simulink model "Base"  (R2013b)
settings: Solver=ode23t  StartTime=0.0  StopTime=1  RelTol=1e-3
undefined symbols (not defined in the file): DiscIntNeverNeededParam
libraries: nesl_utility x11, pe_lib x10, fl_lib x7
Description:
  | Three-Phase PMSM Drive
  | 
  | This example shows a Permanent Magnet Synchronous Machine
  | (PMSM) and inverter sized for use in a typical hybrid vehicle.
  | Here the inverter is connected directly to the vehicle battery, but
  | often there is also a DC-DC converter stage in between. The
  | model can be used to design the PMSM controller, selecting
  | architecture and gains to achieve desired performance. To check
  | the timing of IGBT turn-on and turn-off, the IGBT devices can be
  | directly replaced by more detailed device models from
  | SimElectronics(TM). For complete vehicle modeling, the
  | SimElectronics(R) Servomotor block can be used to abstract the
  | PMSM, inverter and controller with an energy-based model.
  | The Gmin resistor provides a very small conductance to ground
  | that improves the numerical properties of the model when using
  | a variable-step solver.
  | 
  | 
  | Copyright 2008-2013 The MathWorks, Inc.
settings Model: Creator=MathWorks  LastModifiedBy=Eduardo
settings DebuggingCC: SolverPrmCheckMsg=none

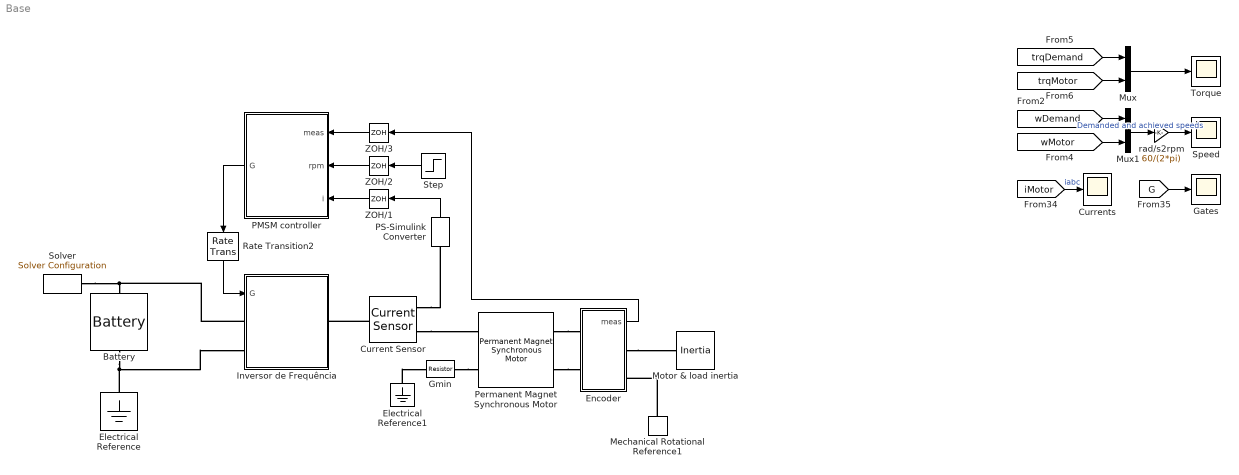
== system Base ==
  Battery : pe_lib/Sources/Battery  Vnom=500 V  AH=14000 hr*A  AH0=7000 hr*A  V1=470 V  AH1=5000 hr*A  R1=0.001 Ohm  R2=inf Ohm  alpha=1  beta=1  G2=0 S  i_Log=off  charge_Log=off  LocalVarNames=|i|charge  LocalVarDescs=|i|Charge state  LocalVarLogging=[0 0]
  Current Sensor : pe_lib/Sensors/Current Sensor  I_Log=off  LocalVarNames=|i_a|i_b|i_c  LocalVarDescs=|i_a|i_b|i_c  LocalVarLogging=[0 0 0]  i_a_Log=off  i_b_Log=off  i_c_Log=off
  Currents : Scope
      settings: TimeRange=1  YMin=-2200  YMax=2200  SaveName=ScopeData5  MaxDataPoints=50000  Decimation=10
  Electrical Reference : fl_lib/Electrical/Electrical Elements/Electrical Reference  i_Log=off  LocalVarNames=|i  LocalVarDescs=|i  LocalVarLogging=0
  Electrical Reference1 : fl_lib/Electrical/Electrical Elements/Electrical Reference  i_Log=off  LocalVarNames=|i  LocalVarDescs=|i  LocalVarLogging=0
  Encoder : Subsystem
  Gates : Scope
      settings: TimeRange=0.01  YMin=-0.1  YMax=1.1  SaveName=ScopeData4  MaxDataPoints=50000  Decimation=10
  Gmin : fl_lib/Electrical/Electrical Elements/Resistor  R=1e9 Ohm  i_Log=off  v_Log=off  LocalVarNames=|i|v  LocalVarDescs=|i|v  LocalVarLogging=[0 0]
  Inversor de Frequência : Subsystem
  Mechanical Rotational Reference1 : fl_lib/Mechanical/Rotational Elements/Mechanical Rotational Reference  t_Log=off  LocalVarNames=|t  LocalVarDescs=|t  LocalVarLogging=0
  Motor & load inertia : fl_lib/Mechanical/Rotational Elements/Inertia  inertia=10 kg*m^2  initial_velocity=0 rpm  t_Log=off  LocalVarNames=|t  LocalVarDescs=|t  LocalVarLogging=0
  Mux : Mux  Inputs=2
  Mux1 : Mux  Inputs=2
  PMSM controller : Subsystem
  PS-Simulink Converter : nesl_utility/PS-Simulink Converter  PhysicalDomain=network_engine_domain  SubClassName=ps_output  LeftPortType=input  RightPortType=output  PseudoPeriodic=off  Frequencies=[]  Unit=A  AffineConversion=off
  Permanent Magnet Synchronous Motor : pe_lib/Machines/Permanent Magnet Rotor/Permanent Magnet Synchronous Motor  nPolePairs=8  pm_flux_linkage=0.03 Wb  stator_param=1  Ld=0.00025 H  Lq=0.00019 H  L0=0.00016 H  Ls=0.0002 H  Lm=0 H  Ms=0 H  Rs=0.013 Ohm  initial_currents=[0, 0, 0] A  axes_param=1  angular_position0=0 deg  LocalVarNames=|i_d|i_q|i_0|v_a|v_b|v_c|i_a|i_b|i_c|torque|angular_velocity|angular_position  LocalVarDescs=|i_d|i_q|i_0|v_a|v_b|v_c|i_a|i_b|i_c|torque|angular_velocity|angular_position  LocalVarLogging=[0 0 0 0 0 0 0 0 0 0 0 0]  rotor_offset=- pi / 2 rad  shift_3ph=[nan, nan, nan] rad  sqrt2OverSqrt3=nan  oneOverSqrt2=nan  twoPiOver3=nan  Lmin=1e-9 H  i_d_Log=off  i_q_Log=off  i_0_Log=off  v_a_Log=off  v_b_Log=off  v_c_Log=off  i_a_Log=off  i_b_Log=off  i_c_Log=off  i_n_Log=off  torque_Log=off  angular_velocity_Log=off  angular_position_Log=off
  Rate Transition2 : RateTransition
  Solver : nesl_utility/Solver Configuration  PhysicalDomain=network_engine_domain  SubClassName=solver  LeftPortType=input  RightPortType=generic  Accelerate=off  Tones=[]  Harmonics=[]  SimulateNoise=off  Profile=off  UseLocalSampling=off  EnableSwitchedLinearOptims=on  FrequencyDomain=off  UseCCode=off  RelTol=0.001  AbsTol=1e-06  MinStep=1e-09  ToWorkspace=off  DoDC=off  ResidualTolerance=1e-9  UseLocalSolver=on  LocalSolverChoice=NE_BACKWARD_EULER_ADVANCER  LocalSolverSampleTime=1e-5  DoFixedCost=on  MaxNonlinIter=3  MaxModeIter=2  LinearAlgebra=Sparse  DelaysMemoryBudget=1024
  Speed : Scope
      settings: YMin=-10  YMax=210  SaveName=ScopeData6  MaxDataPoints=50000  Decimation=10
  Step : Step  Time=0.1  After=200  SampleTime=0
  Torque : Scope
      settings: YMin=-100  YMax=600  SaveName=ScopeData7  MaxDataPoints=50000  Decimation=10
  ZOH/1 : ZeroOrderHold  SampleTime=1e-4
  ZOH/2 : ZeroOrderHold  SampleTime=1e-2
  ZOH/3 : ZeroOrderHold  SampleTime=1e-4
  rad/s2rpm : Gain  Gain=60/(2*pi)
  wires:
  Step/1 -> ZOH/2/1
  PS-Simulink Converter/1 -> ZOH/1/1
  PMSM controller/1(G) -> Rate Transition2/1
  rad/s2rpm/1 -> Speed/1
  [iMotor] -> Currents/1  "iabc"
  [G] -> Gates/1
  Mux1/1 -> rad/s2rpm/1  "Demanded and achieved speeds"
  [wMotor] -> Mux1/2
  [wDemand] -> Mux1/1
  Mux/1 -> Torque/1
  [trqMotor] -> Mux/2
  [trqDemand] -> Mux/1
  ZOH/1/1 -> PMSM controller/3(i)
  ZOH/2/1 -> PMSM controller/2(rpm)
  Encoder/1(meas) -> ZOH/3/1
  ZOH/3/1 -> PMSM controller/1(meas)
  Rate Transition2/1 -> Inversor de Frequência/1(G)
  connections:
  Permanent Magnet Synchronous Motor/RConn1 -- Encoder/LConn1
  Permanent Magnet Synchronous Motor/RConn2 -- Encoder/LConn2
  Encoder/RConn1 -- Motor & load inertia/LConn1
  Mechanical Rotational Reference1/LConn1 -- Encoder/RConn2
  Current Sensor/LConn1 -- Inversor de Frequência/RConn1
  Battery/RConn1 -- Inversor de Frequência/LConn2 -- Electrical Reference/LConn1
  Current Sensor/RConn2 -- Permanent Magnet Synchronous Motor/LConn1
  Current Sensor/RConn1 -- PS-Simulink Converter/LConn1
  Gmin/RConn1 -- Permanent Magnet Synchronous Motor/LConn2
  Electrical Reference1/LConn1 -- Gmin/LConn1
  Solver/RConn1 -- Inversor de Frequência/LConn1 -- Battery/LConn1

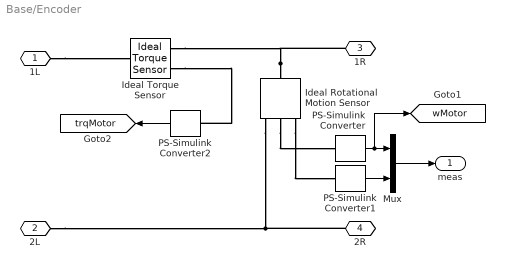
== system Base/Encoder ==
  Ideal Rotational Motion Sensor : fl_lib/Mechanical/Mechanical Sensors/Ideal Rotational Motion Sensor  offset=0 deg  w_Log=off  t_Log=off  phi_Log=off  LocalVarNames=|w|t|phi  LocalVarDescs=|w|t|phi  LocalVarLogging=[0 0 0]
  Ideal Torque Sensor : fl_lib/Mechanical/Mechanical Sensors/Ideal Torque Sensor  w_Log=off  t_Log=off  LocalVarNames=|w|t  LocalVarDescs=|w|t  LocalVarLogging=[0 0]
  Mux : Mux  Inputs=2
  PS-Simulink Converter : nesl_utility/PS-Simulink Converter  PhysicalDomain=network_engine_domain  SubClassName=ps_output  LeftPortType=input  RightPortType=output  PseudoPeriodic=off  Frequencies=[]  Unit=rad/s  AffineConversion=off
  PS-Simulink Converter1 : nesl_utility/PS-Simulink Converter  PhysicalDomain=network_engine_domain  SubClassName=ps_output  LeftPortType=input  RightPortType=output  PseudoPeriodic=off  Frequencies=[]  Unit=rad  AffineConversion=off
  PS-Simulink Converter2 : nesl_utility/PS-Simulink Converter  PhysicalDomain=network_engine_domain  SubClassName=ps_output  LeftPortType=input  RightPortType=output  PseudoPeriodic=off  Frequencies=[]  Unit=N*m  AffineConversion=off
  1L : PMIOPort  Port=1  Side=Left
  2L : PMIOPort  Port=2  Side=Left
  1R : PMIOPort  Port=3  Side=Right
  2R : PMIOPort  Port=4  Side=Right
  meas : Outport
  tag scope: trqMotor=global, wMotor=global
  wires:
  PS-Simulink Converter2/1 -> [trqMotor]
  Mux/1 -> meas/1
  PS-Simulink Converter1/1 -> Mux/2
  PS-Simulink Converter/1 -> [wMotor], Mux/1
  connections:
  Ideal Torque Sensor/RConn2 -- PS-Simulink Converter2/LConn1
  1L/RConn1 -- Ideal Torque Sensor/LConn1
  2R/RConn1 -- 2L/RConn1 -- Ideal Rotational Motion Sensor/RConn1
  Ideal Rotational Motion Sensor/LConn1 -- 1R/RConn1 -- Ideal Torque Sensor/RConn1
  Ideal Rotational Motion Sensor/RConn2 -- PS-Simulink Converter/LConn1
  Ideal Rotational Motion Sensor/RConn3 -- PS-Simulink Converter1/LConn1

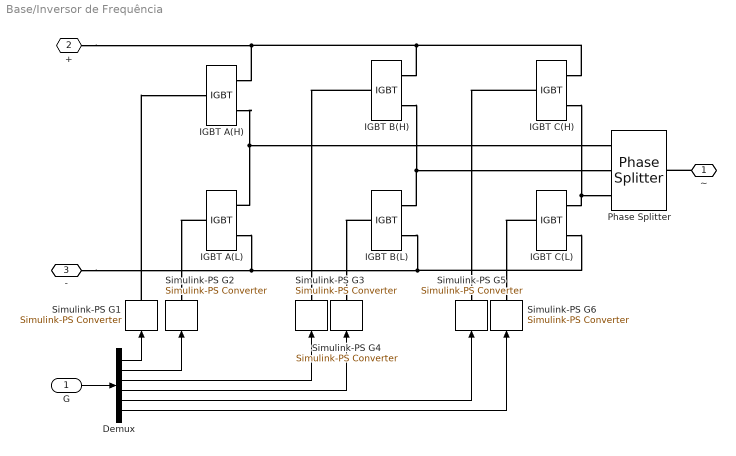
== system Base/Inversor de Frequência ==
  G : Inport
  Demux : Demux  Outputs=6
  IGBT A(H) : pe_lib/Semiconductors/Fundamental Components/IGBT  Vf=0.8 V  Ron=0.001 Ohm  Goff=1e-5 S  Vth=0.5 V  diode_param=2  diode_Vf=0.8 V  diode_Ron=0.001 Ohm  diode_Goff=1e-5 S  diode_C=5e-8 F  diode_iRM=-235 A  diode_iF=300 A  diode_idot=-50 A/us  diode_trr_param=1  diode_trr_factor=3  diode_trr=15 us  diode_Qrr=1.5e+3 s*uA  LocalVarLogging=[]
  IGBT A(L) : pe_lib/Semiconductors/Fundamental Components/IGBT  Vf=0.8 V  Ron=0.001 Ohm  Goff=1e-5 S  Vth=0.5 V  diode_param=2  diode_Vf=0.8 V  diode_Ron=0.001 Ohm  diode_Goff=1e-5 S  diode_C=5e-8 F  diode_iRM=-235 A  diode_iF=300 A  diode_idot=-50 A/us  diode_trr_param=1  diode_trr_factor=3  diode_trr=15 us  diode_Qrr=1.5e+3 s*uA  LocalVarLogging=[]
  IGBT B(H) : pe_lib/Semiconductors/Fundamental Components/IGBT  Vf=0.8 V  Ron=0.001 Ohm  Goff=1e-5 S  Vth=0.5 V  diode_param=2  diode_Vf=0.8 V  diode_Ron=0.001 Ohm  diode_Goff=1e-5 S  diode_C=5e-8 F  diode_iRM=-235 A  diode_iF=300 A  diode_idot=-50 A/us  diode_trr_param=1  diode_trr_factor=3  diode_trr=15 us  diode_Qrr=1.5e+3 s*uA  LocalVarLogging=[]
  IGBT B(L) : pe_lib/Semiconductors/Fundamental Components/IGBT  Vf=0.8 V  Ron=0.001 Ohm  Goff=1e-5 S  Vth=0.5 V  diode_param=2  diode_Vf=0.8 V  diode_Ron=0.001 Ohm  diode_Goff=1e-5 S  diode_C=5e-8 F  diode_iRM=-235 A  diode_iF=300 A  diode_idot=-50 A/us  diode_trr_param=1  diode_trr_factor=3  diode_trr=15 us  diode_Qrr=1.5e+3 s*uA  LocalVarLogging=[]
  IGBT C(H) : pe_lib/Semiconductors/Fundamental Components/IGBT  Vf=0.8 V  Ron=0.001 Ohm  Goff=1e-5 S  Vth=0.5 V  diode_param=2  diode_Vf=0.8 V  diode_Ron=0.001 Ohm  diode_Goff=1e-5 S  diode_C=5e-8 F  diode_iRM=-235 A  diode_iF=300 A  diode_idot=-50 A/us  diode_trr_param=1  diode_trr_factor=3  diode_trr=15 us  diode_Qrr=1.5e+3 s*uA  LocalVarLogging=[]
  IGBT C(L) : pe_lib/Semiconductors/Fundamental Components/IGBT  Vf=0.8 V  Ron=0.001 Ohm  Goff=1e-5 S  Vth=0.5 V  diode_param=2  diode_Vf=0.8 V  diode_Ron=0.001 Ohm  diode_Goff=1e-5 S  diode_C=5e-8 F  diode_iRM=-235 A  diode_iF=300 A  diode_idot=-50 A/us  diode_trr_param=1  diode_trr_factor=3  diode_trr=15 us  diode_Qrr=1.5e+3 s*uA  LocalVarLogging=[]
  Phase Splitter : pe_lib/Connections/Phase Splitter  I_Log=off  i_a_Log=off  i_b_Log=off  i_c_Log=off  LocalVarNames=|I|i_a|i_b|i_c  LocalVarDescs=|I|i_a|i_b|i_c  LocalVarLogging=[0 0 0 0]
  Simulink-PS G{1..6} (6 alike) : nesl_utility/Simulink-PS Converter  PhysicalDomain=network_engine_domain  SubClassName=ps_input  LeftPortType=input  RightPortType=output  PseudoPeriodic=off  Frequencies=[]  NoiseDistribution=none  NoiseParameters=[]  Unit=1  AffineConversion=off  InputFiltering=off  SimscapeFilterOrder=1  InputFilterTimeConstant=1e-6  UdotUserProvided=0
  ~ : PMIOPort  Tag=PMCPort  Port=1  Side=Right
  + : PMIOPort  Tag=PMCPort  Port=2  Side=Left
  - : PMIOPort  Tag=PMCPort  Port=3  Side=Left
  wires:
  Demux/6 -> Simulink-PS G6/1
  Demux/5 -> Simulink-PS G5/1
  Demux/4 -> Simulink-PS G4/1
  Demux/3 -> Simulink-PS G3/1
  Demux/2 -> Simulink-PS G2/1
  G/1 -> Demux/1
  Demux/1 -> Simulink-PS G1/1
  connections:
  IGBT C(L)/LConn1 -- Simulink-PS G6/RConn1
  IGBT C(H)/LConn1 -- Simulink-PS G5/RConn1
  IGBT B(L)/LConn1 -- Simulink-PS G4/RConn1
  IGBT B(H)/LConn1 -- Simulink-PS G3/RConn1
  IGBT A(L)/LConn1 -- Simulink-PS G2/RConn1
  -/RConn1 -- IGBT A(L)/RConn2 -- IGBT C(L)/RConn2 -- IGBT B(L)/RConn2
  IGBT A(H)/RConn2 -- IGBT A(L)/RConn1 -- Phase Splitter/RConn1
  IGBT B(L)/RConn1 -- IGBT B(H)/RConn2 -- Phase Splitter/RConn2
  IGBT C(L)/RConn1 -- IGBT C(H)/RConn2 -- Phase Splitter/RConn3
  +/RConn1 -- IGBT A(H)/RConn1 -- IGBT C(H)/RConn1 -- IGBT B(H)/RConn1
  ~/RConn1 -- Phase Splitter/LConn1
  Simulink-PS G1/RConn1 -- IGBT A(H)/LConn1

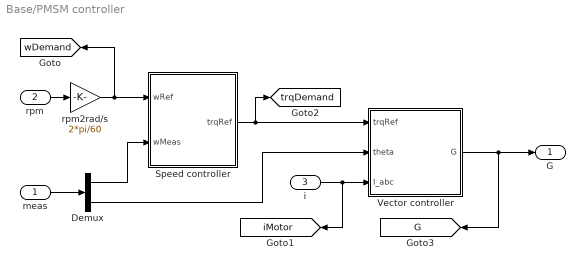
== system Base/PMSM controller ==
  meas : Inport
  rpm : Inport  Port=2
  i : Inport  Port=3
  Demux : Demux  Outputs=2
  Speed controller : Subsystem  mask(P+I motor speed controller){Kp=10000, Ki=10000, trqMax=500, ts=1e-2}
      mask prompts: Kp "Proportional gain (Nm/(rad/s))"; Ki "Integral gain (Nm/rad)"; trqMax "Maximum torque demand"; ts "Sample time"
      mask help: Inputs wRef and wMeas are the demanded rotor speed and measured rotor speed in rad/s. The controller output is a torque demand in Nm.
  Vector controller : Subsystem  mask(Vector controller){Np=6, lambda=0.03, h=1}
      mask prompts: Np "Number of pole pairs, p"; lambda "Flux linkage from rotor permanent magnet"; h "Current hysteresis (A)"
  rpm2rad/s : Gain  Gain=2*pi/60
  G : Outport
  tag scope: G=global, iMotor=global, trqDemand=global, wDemand=global
  wires:
  Vector controller/1(G) -> G/1, [G]
  Speed controller/1(trqRef) -> [trqDemand], Vector controller/1(trqRef)
  i/1 -> [iMotor], Vector controller/3(I_abc)
  rpm/1 -> rpm2rad/s/1
  rpm2rad/s/1 -> Speed controller/1(wRef), [wDemand]
  meas/1 -> Demux/1
  Demux/1 -> Speed controller/2(wMeas)
  Demux/2 -> Vector controller/2(theta)

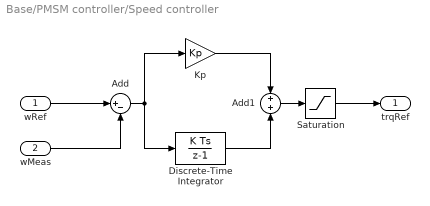
== system Base/PMSM controller/Speed controller ==
  wRef : Inport
  wMeas : Inport  Port=2
  Add : Sum  Inputs=|+-
  Add1 : Sum
  Discrete-Time Integrator : DiscreteIntegrator  gainval=Ki  SampleTime=ts  LimitOutput=on  UpperSaturationLimit=trqMax  LowerSaturationLimit=-trqMax  ICPrevOutput=DiscIntNeverNeededParam  ICPrevScaledInput=DiscIntNeverNeededParam
  Kp : Gain  Gain=Kp
  Saturation : Saturate  UpperLimit=trqMax  LowerLimit=-trqMax
  trqRef : Outport
  wires:
  wRef/1 -> Add/1
  Add1/1 -> Saturation/1
  Kp/1 -> Add1/1
  Discrete-Time Integrator/1 -> Add1/2
  wMeas/1 -> Add/2
  Saturation/1 -> trqRef/1
  Add/1 -> Kp/1, Discrete-Time Integrator/1

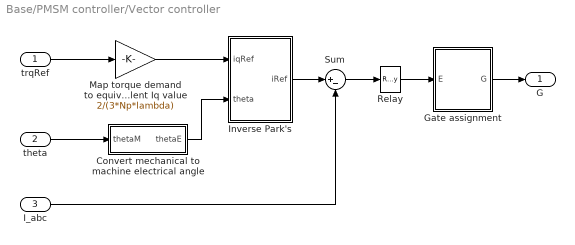
== system Base/PMSM controller/Vector controller ==
  trqRef : Inport
  theta : Inport  Port=2
  I_abc : Inport  Port=3
  Convert mechanical to machine electrical angle : Subsystem
  Gate assignment : Subsystem
  Inverse Park's : Subsystem
  Map torque demand to equivalent Iq value : Gain  Gain=2/(3*Np*lambda)  SaturateOnIntegerOverflow=on  OutDataTypeStr=Inherit: Same as input  ParamDataTypeStr=Inherit: Same as input
  Relay : Relay  OnSwitchValue=h/2  OffSwitchValue=-h/2
  Sum : Sum  Inputs=|+-  SaturateOnIntegerOverflow=on  InputSameDT=on  OutDataTypeStr=Inherit: Same as first input
  G : Outport
  wires:
  Convert mechanical to machine electrical angle/1(thetaE) -> Inverse Park's/2(theta)
  theta/1 -> Convert mechanical to machine electrical angle/1(thetaM)
  Map torque demand to equivalent Iq value/1 -> Inverse Park's/1(iqRef)
  I_abc/1 -> Sum/2
  trqRef/1 -> Map torque demand to equivalent Iq value/1
  Inverse Park's/1(iRef) -> Sum/1
  Sum/1 -> Relay/1
  Relay/1 -> Gate assignment/1(E)
  Gate assignment/1(G) -> G/1

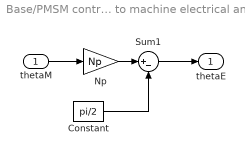
== system Base/PMSM controller/Vector controller/Convert mechanical to machine electrical angle ==
  thetaM : Inport
  Constant : Constant  Value=pi/2
  Np : Gain  Gain=Np  SaturateOnIntegerOverflow=on  OutDataTypeStr=Inherit: Same as input  ParamDataTypeStr=Inherit: Same as input
  Sum1 : Sum  Inputs=|+-
  thetaE : Outport
  wires:
  Constant/1 -> Sum1/2
  thetaM/1 -> Np/1
  Np/1 -> Sum1/1
  Sum1/1 -> thetaE/1

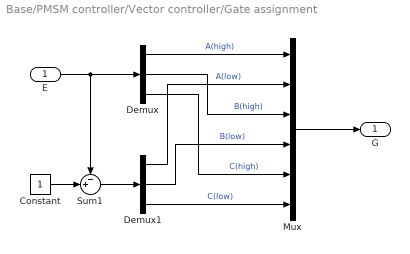
== system Base/PMSM controller/Vector controller/Gate assignment ==
  E : Inport
  Constant : Constant
  Demux : Demux  Outputs=3
  Demux1 : Demux  Outputs=3
  Mux : Mux  Inputs=6
  Sum1 : Sum  Inputs=-+|  SaturateOnIntegerOverflow=on  InputSameDT=on  OutDataTypeStr=Inherit: Same as first input
  G : Outport
  wires:
  Demux/3 -> Mux/5  "C(high)"
  Demux1/3 -> Mux/6  "C(low)"
  Mux/1 -> G/1
  Sum1/1 -> Demux1/1
  E/1 -> Sum1/1, Demux/1
  Constant/1 -> Sum1/2
  Demux/1 -> Mux/1  "A(high)"
  Demux/2 -> Mux/3  "B(high)"
  Demux1/2 -> Mux/4  "B(low)"
  Demux1/1 -> Mux/2  "A(low)"

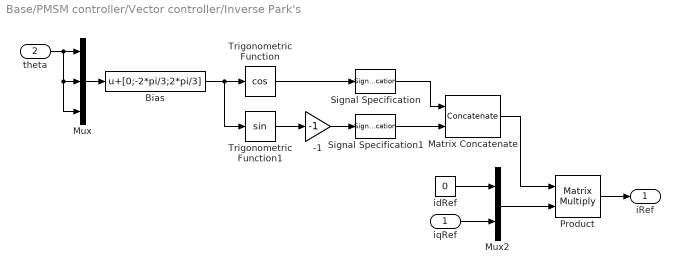
== system Base/PMSM controller/Vector controller/Inverse Park's ==
  iqRef : Inport
  theta : Inport  Port=2
  -1 : Gain  Gain=-1  SaturateOnIntegerOverflow=on  OutDataTypeStr=Inherit: Same as input  ParamDataTypeStr=Inherit: Same as input
  Bias : Bias  Bias=[0;-2*pi/3;2*pi/3]
  Matrix Concatenate : Concatenate  Mode=Multidimensional array  ConcatenateDimension=2
  Mux : Mux  Inputs=3
  Mux2 : Mux  Inputs=2
  Product : Product  Multiplication=Matrix(*)  RndMeth=Zero
  Signal Specification : SignalSpecification  Dimensions=[3 1]
  Signal Specification1 : SignalSpecification  Dimensions=[3 1]
  Trigonometric Function : Trigonometry  Operator=cos
  Trigonometric Function1 : Trigonometry
  idRef : Constant  Value=0
  iRef : Outport  InitialOutput=0
  wires:
  Mux/1 -> Bias/1
  Matrix Concatenate/1 -> Product/1
  Mux2/1 -> Product/2
  iqRef/1 -> Mux2/2
  idRef/1 -> Mux2/1
  Signal Specification/1 -> Matrix Concatenate/1
  Signal Specification1/1 -> Matrix Concatenate/2
  Trigonometric Function1/1 -> -1/1
  Bias/1 -> Trigonometric Function/1, Trigonometric Function1/1
  theta/1 -> Mux/3, Mux/2, Mux/1
  Product/1 -> iRef/1
  Trigonometric Function/1 -> Signal Specification/1
  -1/1 -> Signal Specification1/1
